simulink model "untitled"  (R2021a)
settings: Solver=VariableStepAuto  StartTime=0.0  StopTime=inf  RelTol=1e-3
settings Model: Creator=thana  LastModifiedBy=thana

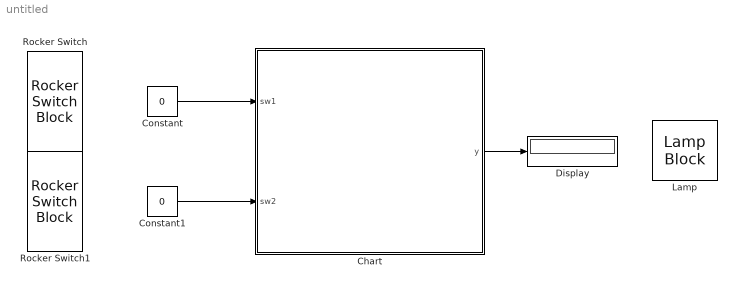
== system untitled ==
  Chart : Stateflow chart  TreatAsAtomicUnit=on
  Constant : Constant  Value=0
  Constant1 : Constant  Value=0
  Display : Display
  Lamp : LampBlock
  Rocker Switch : RockerSwitchBlock
      settings: Values={{'Off', 'On'}, [0 1]}
  Rocker Switch1 : RockerSwitchBlock
      settings: Values={{'Off', 'On'}, [0 1]}
  wires:
  Constant/1 -> Chart/1(sw1)
  Constant1/1 -> Chart/2(sw2)
  Chart/1(y) -> Display/1

== stateflow chart untitled/Chart ==
  state Off
    during:
    y = 0
  state On
    during:
    y = 0
  state Play
    during:
    y = 1
  (default) -> Off
  Off -> On : [sw1 == 1]{y = 0}
  On -> Off [order 2] : [sw1 == 0]{y = 0}
  Play -> Off [order 1] : [sw1 == 0]{y = 0}
  Play -> On [order 2] : [sw2 == 0 && sw1 == 1]{y = 0}
  On -> Play [order 1] : [sw2 == 1]{y = 1}
  data: sw1 input; y output; sw2 input
